simulink model "secondordersys"  (R2015a)
settings: Solver=ode45  StartTime=0.0  StopTime=10.0  RelTol=1e-3
settings Model: Creator=LENOVO  LastModifiedBy=LENOVO

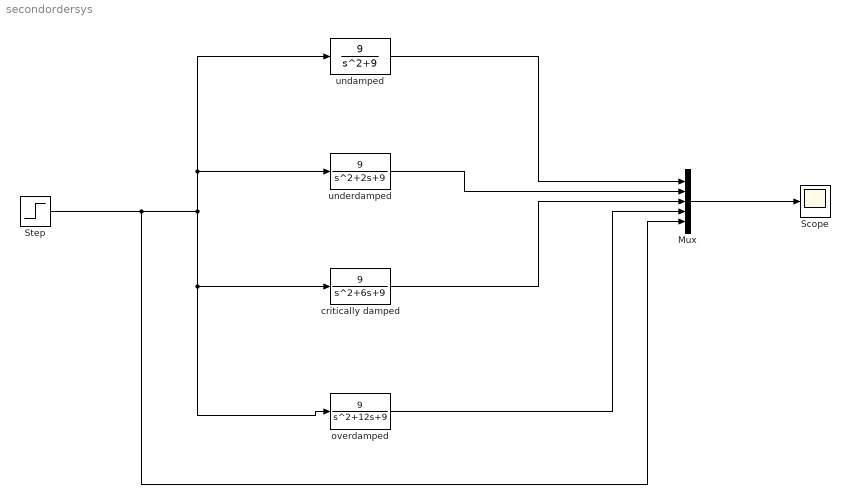
== system secondordersys ==
  Mux : Mux  Inputs=5
  Scope : Scope
      settings: ShowLegends=on
  Step : Step  Time=0  SampleTime=0
  critically damped : TransferFcn  Numerator=[9]  Denominator=[1 6 9]
  overdamped : TransferFcn  Numerator=[9]  Denominator=[1 12 9]
  undamped : TransferFcn  Numerator=[9]  Denominator=[1 0 9]
  underdamped : TransferFcn  Numerator=[9]  Denominator=[1 2 9]
  wires:
  undamped/1 -> Mux/1
  underdamped/1 -> Mux/2
  critically damped/1 -> Mux/3
  overdamped/1 -> Mux/4
  Step/1 -> Mux/5, undamped/1, underdamped/1, critically damped/1, overdamped/1
  Mux/1 -> Scope/1
